simulink subsystem "subref_minimize_saturation"  (R2024b)
settings: Solver=VariableStepAuto  StartTime=0.0  StopTime=10.0  RelTol=1e-3
libraries: simulink x1
settings Model: Creator=CETCA  LastModifiedBy=CETCA

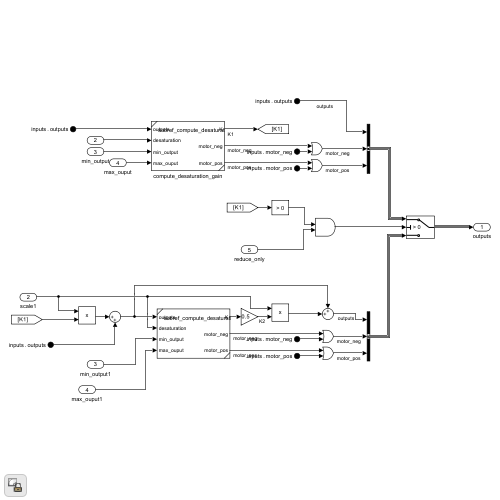
[thumbnail: Simulink's stored preview of the top-level diagram]
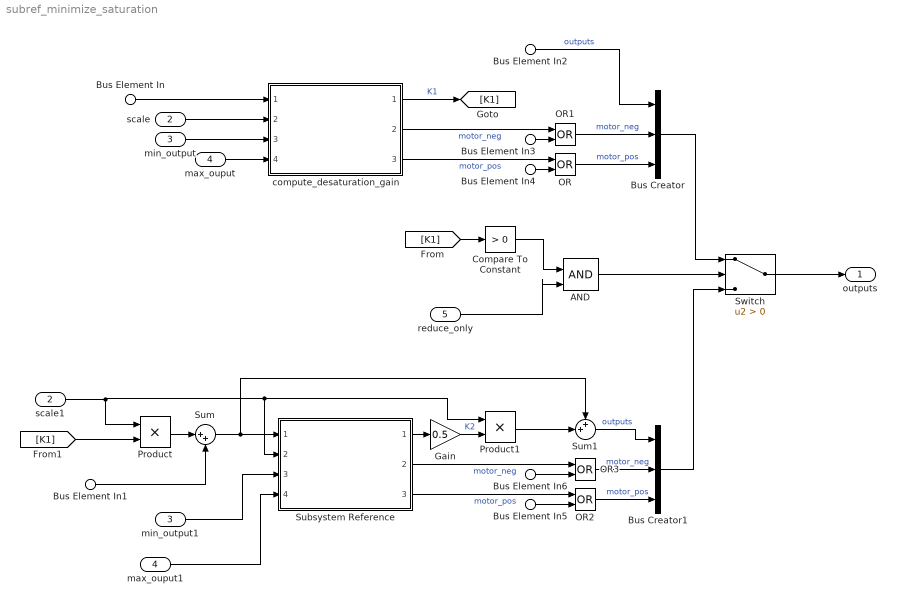
== system subref_minimize_saturation ==
  Bus Element In : Inport  PortName=inputs  Element=outputs
  Bus Element In1 : Inport  PortName=inputs  Element=outputs
  Bus Element In2 : Inport  PortName=inputs  Element=outputs
  Bus Element In3 : Inport  PortName=inputs  Element=motor_neg
  Bus Element In6 : Inport  PortName=inputs  Element=motor_neg
  Bus Element In4 : Inport  PortName=inputs  Element=motor_pos
  Bus Element In5 : Inport  PortName=inputs  Element=motor_pos
  scale : Inport  Port=2
  min_output : Inport  Port=3
  max_ouput : Inport  Port=4
  reduce_only : Inport  Port=5
  AND : Logic  IconShape=distinctive  AllPortsSameDT=off  OutDataTypeStr=boolean
  Bus Creator : BusCreator  Inputs=3
  Bus Creator1 : BusCreator  Inputs=3
  Compare To Constant : simulink/Logic and Bit Operations/Compare To Constant  relop=>  const=0  OutDataTypeStr=boolean
  Gain : Gain  Gain=0.5
  OR{,1..3} (4 alike) : Logic  Operator=OR  IconShape=distinctive  AllPortsSameDT=off  OutDataTypeStr=boolean
  Product : Product
  Product1 : Product
  Subsystem Reference : Subsystem  ReferencedSubsystem=subref_compute_desaturation_gain
  Sum : Sum  Inputs=|++
  Sum1 : Sum  Inputs=++|
  Switch : Switch  Criteria=u2 > Threshold  SaturateOnIntegerOverflow=off  InputSameDT=off
  compute_desaturation_gain : Subsystem  ReferencedSubsystem=subref_compute_desaturation_gain
  max_ouput1 : InportShadow  Port=4
  min_output1 : InportShadow  Port=3
  scale1 : InportShadow  Port=2
  outputs : Outport
  wires:
  Bus Element In/1 -> compute_desaturation_gain/1
  scale/1 -> compute_desaturation_gain/2
  min_output/1 -> compute_desaturation_gain/3
  max_ouput/1 -> compute_desaturation_gain/4
  scale1/1 -> Product/1, Product1/1, Subsystem Reference/2
  Product/1 -> Sum/1
  Bus Element In1/1 -> Sum/2
  reduce_only/1 -> AND/2
  compute_desaturation_gain/1 -> [K1]  "K1"
  [K1] -> Compare To Constant/1
  Compare To Constant/1 -> AND/1
  AND/1 -> Switch/2
  [K1] -> Product/2
  Sum/1 -> Sum1/1, Subsystem Reference/1
  min_output1/1 -> Subsystem Reference/3
  max_ouput1/1 -> Subsystem Reference/4
  Bus Element In2/1 -> Bus Creator/1  "outputs"
  OR/1 -> Bus Creator/3  "motor_pos"
  Bus Creator/1 -> Switch/1
  Subsystem Reference/1 -> Gain/1
  Gain/1 -> Product1/2  "K2"
  Product1/1 -> Sum1/2
  Sum1/1 -> Bus Creator1/1  "outputs"
  OR3/1 -> Bus Creator1/2  "motor_neg"
  OR2/1 -> Bus Creator1/3  "motor_pos"
  Bus Creator1/1 -> Switch/3
  Switch/1 -> outputs/1
  OR1/1 -> Bus Creator/2  "motor_neg"
  compute_desaturation_gain/2 -> OR1/1  "motor_neg"
  compute_desaturation_gain/3 -> OR/1  "motor_pos"
  Bus Element In3/1 -> OR1/2
  Bus Element In4/1 -> OR/2
  Subsystem Reference/3 -> OR2/1  "motor_pos"
  Bus Element In5/1 -> OR2/2
  Subsystem Reference/2 -> OR3/1  "motor_neg"
  Bus Element In6/1 -> OR3/2
